simulink model "hill_analytical_optimise_compare"  (R2022b)
settings: Solver=VariableStepAuto  StartTime=0.0  StopTime=8000  RelTol=1e-3
settings Model: Creator=u1473578  LastModifiedBy=u1473578

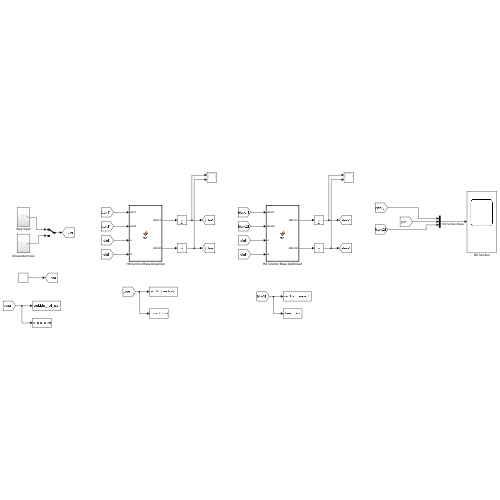
[thumbnail: Simulink's stored preview of the top-level diagram]
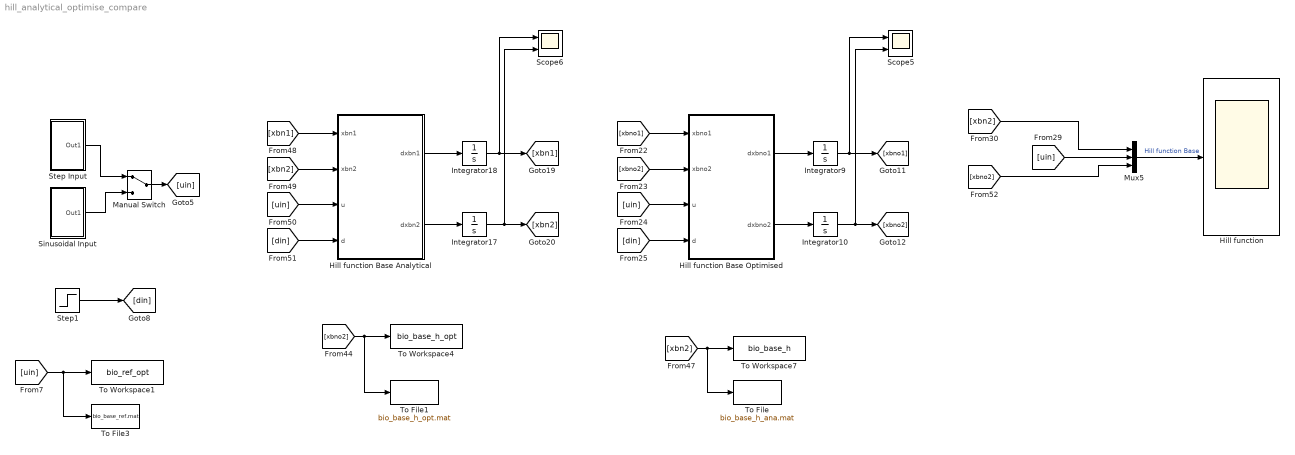
== system hill_analytical_optimise_compare ==
  Hill function : Scope
  Hill function Base Analytical : MATLAB Function  TreatAsAtomicUnit=on
  Hill function Base Optimised : MATLAB Function  TreatAsAtomicUnit=on
  Integrator{9..10,17..18} (4 alike) : Integrator
  Manual Switch : ManualSwitch
  Mux5 : Mux  Inputs=3
  Scope5 : Scope  NumInputPorts=2
  Scope6 : Scope  NumInputPorts=2
  Sinusoidal Input : Subsystem
  Step Input : Subsystem
  Step1 : Step  Time=3000-0*1000  After=1*0.05*(-5e-4)  SampleTime=0
  To File : ToFile  Filename=bio_base_h_ana.mat  MatrixName=xbna2  SaveFormat=Timeseries
  To File1 : ToFile  Filename=bio_base_h_opt.mat  MatrixName=xbno2  SaveFormat=Timeseries
  To File3 : ToFile  Filename=bio_base_ref.mat  MatrixName=uref  SaveFormat=Timeseries
  To Workspace1 : ToWorkspace  VariableName=bio_ref_opt  SaveFormat=Timeseries  SampleTime=-1
  To Workspace4 : ToWorkspace  VariableName=bio_base_h_opt  SaveFormat=Timeseries  SampleTime=-1
  To Workspace7 : ToWorkspace  VariableName=bio_base_h  SaveFormat=Timeseries  SampleTime=-1
  wires:
  Hill function Base Analytical/2(dxbn2) -> Integrator17/1
  Integrator18/1 -> Scope6/1, [xbn1]
  [xbno2] -> Mux5/3
  [uin] -> Mux5/2
  Step1/1 -> [din]
  [uin] -> Hill function Base Analytical/3(u)
  [xbn2] -> To File/1, To Workspace7/1
  Integrator17/1 -> Scope6/2, [xbn2]
  [xbn1] -> Hill function Base Analytical/1(xbn1)
  [xbn2] -> Hill function Base Analytical/2(xbn2)
  Hill function Base Analytical/1(dxbn1) -> Integrator18/1
  [uin] -> Hill function Base Optimised/3(u)
  [din] -> Hill function Base Analytical/4(d)
  [xbno2] -> To File1/1, To Workspace4/1
  Hill function Base Optimised/1(dxbno1) -> Integrator9/1
  [uin] -> To File3/1, To Workspace1/1
  [xbno2] -> Hill function Base Optimised/2(xbno2)
  [xbno1] -> Hill function Base Optimised/1(xbno1)
  [xbn2] -> Mux5/1
  Mux5/1 -> Hill function/1  "Hill function Base"
  Step Input/1(Out1) -> Manual Switch/1
  [din] -> Hill function Base Optimised/4(d)
  Hill function Base Optimised/2(dxbno2) -> Integrator10/1
  Integrator10/1 -> Scope5/2, [xbno2]
  Manual Switch/1 -> [uin]
  Integrator9/1 -> Scope5/1, [xbno1]
  Sinusoidal Input/1(Out1) -> Manual Switch/2

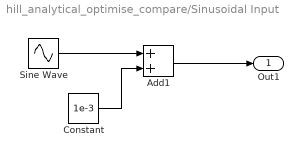
== system hill_analytical_optimise_compare/Sinusoidal Input ==
  Add1 : Sum
  Constant : Constant  Value=1e-3
  Sine Wave : Sin  Amplitude=1e-3  Frequency=10/6000  Phase=2800-150  SampleTime=0
  Out1 : Outport
  wires:
  Sine Wave/1 -> Add1/1
  Constant/1 -> Add1/2
  Add1/1 -> Out1/1

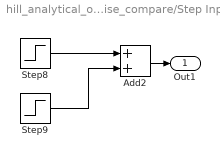
== system hill_analytical_optimise_compare/Step Input ==
  Add2 : Sum
  Step8 : Step  Time=0  After=0  SampleTime=0
  Step9 : Step  Time=1000  After=1e-3  SampleTime=0
  Out1 : Outport
  wires:
  Step9/1 -> Add2/2
  Step8/1 -> Add2/1
  Add2/1 -> Out1/1

== matlab function hill_analytical_optimise_compare/Hill function Base Optimised ==
  data: xbno1 input; xbno2 input; u input; dxbno1 output; dxbno2 output; d input
function [dxbno1,dxbno2] = fcn(xbno1,xbno2,u,d)

% x1 = X
% x2 = Z

gamma = 1;
c = gamma;
%% Derived Parameters through two-point matching (Inhibition Type 1)
% Kx = 0.002;
% Kz = 0.08;
% 
% % per minutes
% delta_x = 0.0005;
% delta_z = 0.02;
% 
% alpha_x = 2e-8;
% alpha_z = 1e-4;
% 
% bs = -5e-3;

%% Derived Parameters through two-point matching (Inhibition Type 2)
% Kx = 0.002; % analytic
Kx = 0.0022; % optimise
% Kz = 0.08; % analytic
Kz = 0.1896; % optimise

% per minutes
delta_x = 0.0005;
delta_z = 0.02;

% alpha_x = 0.005; % analytic
alpha_x = 0.0051; % optimise
% alpha_z = 1e-4; % analytic
alpha_z = 2e-4; % optimise

bs = -5e-3;


%% Matthew's Parameters (Inhibiition Type 2)
% Kx = sqrt(0.05);
% Kz = sqrt(0.05);
% 
% % per minutes
% delta_x = 0.5;
% delta_z = 0.5;
% 
% alpha_x = 0.5;
% alpha_z = 0.5;
% 
% bs = -0.5;

%% ODE

% Inhibition Type 1
% dxbn1 = c*u + ((alpha_x)/(Kx^2 + xbn2^2) + bs) - delta_x*xbn1;

% Inhibition Type 2
dxbno1 = c*u + ((alpha_x*Kx^2)/(Kx^2 + xbno2^2) + bs) - delta_x*xbno1;

dxbno2 = (alpha_z*xbno1^2/(Kz^2 + xbno1^2)) - delta_z*xbno2 + 1*d;

== matlab function hill_analytical_optimise_compare/Hill function Base Analytical ==
  data: xbn1 input; xbn2 input; u input; dxbn1 output; dxbn2 output; d input
function [dxbn1,dxbn2] = fcn(xbn1,xbn2,u,d)

% x1 = X
% x2 = Z

gamma = 1;
c = gamma;
%% Derived Parameters through two-point matching (Inhibition Type 1)
% Kx = 0.002;
% Kz = 0.08;
% 
% % per minutes
% delta_x = 0.0005;
% delta_z = 0.02;
% 
% alpha_x = 2e-8;
% alpha_z = 1e-4;
% 
% bs = -5e-3;

%% Derived Parameters through two-point matching (Inhibition Type 2)
Kx = 0.002;
Kz = 0.08;

% per minutes
delta_x = 0.0005;
delta_z = 0.02;

alpha_x = 0.005;
alpha_z = 1e-4;

bs = -5e-3;


%% Matthew's Parameters (Inhibiition Type 2)
% Kx = sqrt(0.05);
% Kz = sqrt(0.05);
% 
% % per minutes
% delta_x = 0.5;
% delta_z = 0.5;
% 
% alpha_x = 0.5;
% alpha_z = 0.5;
% 
% bs = -0.5;

%% ODE

% Inhibition Type 1
% dxbn1 = c*u + ((alpha_x)/(Kx^2 + xbn2^2) + bs) - delta_x*xbn1;

% Inhibition Type 2
dxbn1 = c*u + ((alpha_x*Kx^2)/(Kx^2 + xbn2^2) + bs) - delta_x*xbn1;

dxbn2 = (alpha_z*xbn1^2/(Kz^2 + xbn1^2)) - delta_z*xbn2 + 1*d;
